simulink model "SpeedControl"  (Simulink 7.7)
settings: Solver=ode45  StartTime=0.0  StopTime=5  FixedStep=1e-6  RelTol=1e-3
values from neighbouring files (symbols this model uses):
  detaGND = 1.6    [all.mat]
  Ts = 0.01    [all.mat]
  WnGND = 3.5    [all.mat]
libraries: simulink x1
settings Model: Creator=Administrator  LastModifiedBy=Administrator

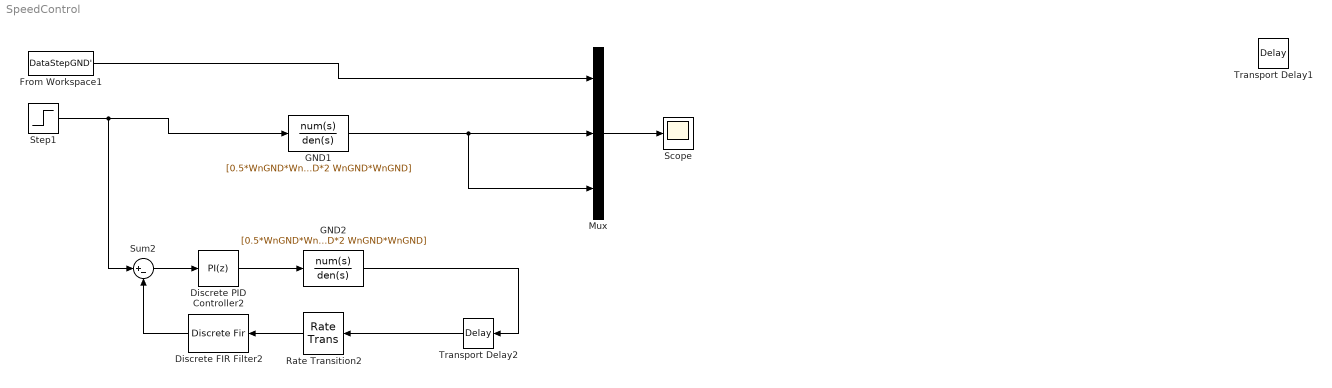
== system SpeedControl ==
  Discrete FIR Filter2 : DiscreteFir  NumCoeffs=[0.333 0.333 0.333]
  Discrete PID Controller2 : simulink/Continuous/PID Controller  SystemSampleTime=-1  Controller=PI  TimeDomain=Discrete-time  SampleTime=Ts  IntegratorMethod=Forward Euler  FilterMethod=Forward Euler  Form=Parallel  P=4  I=6  D=0.0364210490711884  N=189.887708441779  InitialConditionSource=internal  InitialConditionForIntegrator=0  InitialConditionForFilter=0  ExternalReset=none  LimitOutput=on  UpperSaturationLimit=1000  LowerSaturationLimit=-1000  LinearizeAsGain=off  AntiWindupMode=clamping  Kb=1  TrackingMode=off  Kt=1  PParamMin=[]  PParamMax=[]  IParamMin=[]  IParamMax=[]  DParamMin=[]  DParamMax=[]  NParamMin=[]  NParamMax=[]  KbParamMin=[]  KbParamMax=[]  KtParamMin=[]  KtParamMax=[]  POutMin=[]  POutMax=[]  IOutMin=[]  IOutMax=[]  DOutMin=[]  DOutMax=[]  NOutMin=[]  NOutMax=[]  KbOutMin=[]  KbOutMax=[]  KtOutMin=[]  KtOutMax=[]  IntegratorOutMin=[]  IntegratorOutMax=[]  FilterOutMin=[]  FilterOutMax=[]  SumOutMin=[]  SumOutMax=[]  SumI1OutMin=[]  SumI1OutMax=[]  SumI2OutMin=[]  SumI2OutMax=[]  SumI3OutMin=[]  SumI3OutMax=[]  SumDOutMin=[]  SumDOutMax=[]  SaturationOutMin=[]  SaturationOutMax=[]  IntegratorContinuousStateAttributes=''  IntegratorStateMustResolveToSignalObject=off  IntegratorRTWStateStorageClass=Auto  FilterContinuousStateAttributes=''  FilterStateMustResolveToSignalObject=off  FilterRTWStateStorageClass=Auto
  From Workspace1 : FromWorkspace  VariableName=DataStepGND'  SampleTime=0.0067*2
  GND1 : TransferFcn  Numerator=[0.5*WnGND*WnGND]  Denominator=[1 WnGND*detaGND*2 WnGND*WnGND]
  GND2 : TransferFcn  Numerator=[0.5*WnGND*WnGND]  Denominator=[1 WnGND*detaGND*2 WnGND*WnGND]
  Mux : Mux  Inputs=3
  Rate Transition2 : RateTransition  OutPortSampleTime=Ts
  Scope : Scope
      settings: YMin=0  YMax=275
  Step1 : Step  Time=5  Before=250  After=250  SampleTime=Ts
  Sum2 : Sum  Inputs=|+-  SampleTime=Ts
  Transport Delay1 : TransportDelay  DelayTime=0.005
  Transport Delay2 : TransportDelay  DelayTime=0.005
  wires:
  Mux/1 -> Scope/1
  ? -> Transport Delay1/1
  Discrete PID Controller2/1 -> GND2/1
  Sum2/1 -> Discrete PID Controller2/1
  Rate Transition2/1 -> Discrete FIR Filter2/1
  Discrete FIR Filter2/1 -> Sum2/2
  Transport Delay2/1 -> Rate Transition2/1
  GND2/1 -> Transport Delay2/1
  From Workspace1/1 -> Mux/1
  Step1/1 -> GND1/1, Sum2/1
  GND1/1 -> Mux/2, Mux/3
